simulink model "midterm_block_diagram"  (R2025b)
settings: Solver=VariableStepAuto  StartTime=0.0  StopTime=10.0  RelTol=1e-3
model workspace (MAT data in the model file):
  L_hover = 1
  M_hover = 1
  T_hover = 1
  k1 = 1
  k2 = 1
  k3 = 1
  k4 = 1
  k5 = 1
  x_ref = 1
  y_ref = 1
  z_ref = 1
values from neighbouring files (symbols this model uses):
  K = lqr(A, B, Q, R)    [altitude_control.m]    (also in forward_position_control.m; kalman_filtering.m = P_minus * Cd' / S; lateral_position_control.m; matlab.mat = [0.000497379272644 -0.00135191457606 0.000112708319641 -7.98)
settings Model: Creator=toby0830  LastModifiedBy=tobys

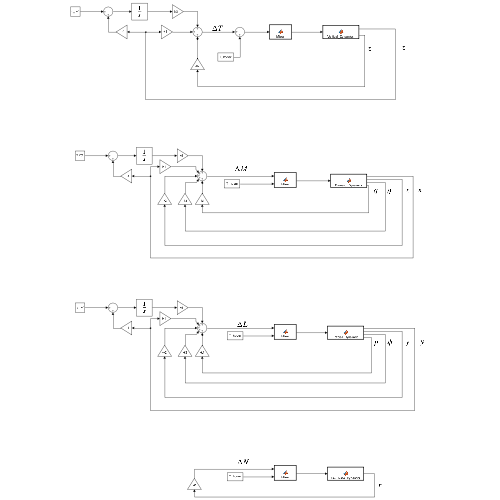
[thumbnail: Simulink's stored preview of the top-level diagram]
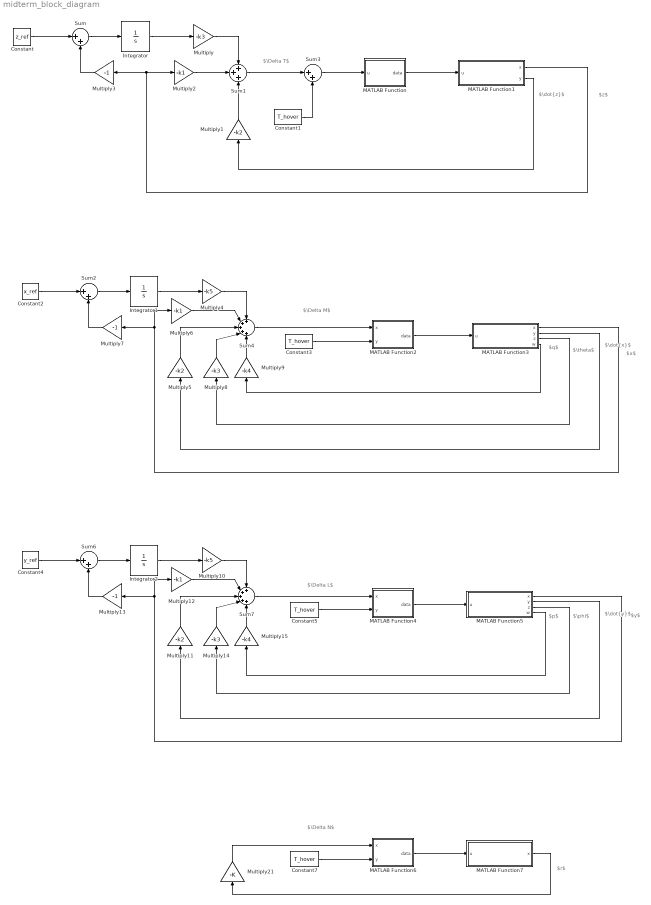
== system midterm_block_diagram ==
  note: $z$
  note: $\dot{x}$
  note: $x$
  note: $\theta$
  note: $q$
  note: $\Delta M$
  note: $\dot{z}$
  note: $\dot{y}$
  note: $y$
  note: $p$
  note: $\Delta L$
  note: $\phi$
  note: $r$
  note: $\Delta N$
  note: $\Delta T$
  Constant : Constant  Value=z_ref
  Constant{1,3,5,7} (4 alike) : Constant  Value=T_hover
  Constant2 : Constant  Value=x_ref
  Constant4 : Constant  Value=y_ref
  Integrator : Integrator
  Integrator1 : Integrator
  Integrator2 : Integrator
  MATLAB Function : MATLAB Function  TreatAsAtomicUnit=on
  MATLAB Function1 : MATLAB Function  TreatAsAtomicUnit=on
  MATLAB Function2 : MATLAB Function  TreatAsAtomicUnit=on
  MATLAB Function3 : MATLAB Function  TreatAsAtomicUnit=on
  MATLAB Function4 : MATLAB Function  TreatAsAtomicUnit=on
  MATLAB Function5 : MATLAB Function  TreatAsAtomicUnit=on
  MATLAB Function6 : MATLAB Function  TreatAsAtomicUnit=on
  MATLAB Function7 : MATLAB Function  TreatAsAtomicUnit=on
  Multiply : Gain  Gain=-k3
  Multiply1 : Gain  Gain=-k2
  Multiply10 : Gain  Gain=-k5
  Multiply11 : Gain  Gain=-k2
  Multiply12 : Gain  Gain=-k1
  Multiply13 : Gain  Gain=-1
  Multiply14 : Gain  Gain=-k3
  Multiply15 : Gain  Gain=-k4
  Multiply2 : Gain  Gain=-k1
  Multiply21 : Gain  Gain=-K
  Multiply3 : Gain  Gain=-1
  Multiply4 : Gain  Gain=-k5
  Multiply5 : Gain  Gain=-k2
  Multiply6 : Gain  Gain=-k1
  Multiply7 : Gain  Gain=-1
  Multiply8 : Gain  Gain=-k3
  Multiply9 : Gain  Gain=-k4
  Sum{,2..3,6} (4 alike) : Sum  Inputs=|++
  Sum1 : Sum  Inputs=+++
  Sum4 : Sum  Inputs=+++++
  Sum7 : Sum  Inputs=+++++
  wires:
  Constant/1 -> Sum/1
  Sum/1 -> Integrator/1
  Integrator/1 -> Multiply/1
  Multiply/1 -> Sum1/1
  Sum1/1 -> Sum3/1
  Constant1/1 -> Sum3/2
  Sum3/1 -> MATLAB Function/1(u)
  MATLAB Function/1(data) -> MATLAB Function1/1(u)
  MATLAB Function1/2(y) -> Multiply1/1
  MATLAB Function1/1(x) -> Multiply3/1, Multiply2/1
  Multiply2/1 -> Sum1/2
  Multiply1/1 -> Sum1/3
  Multiply3/1 -> Sum/2
  Multiply4/1 -> Sum4/1
  MATLAB Function3/2(y) -> Multiply5/1
  Constant2/1 -> Sum2/1
  Multiply7/1 -> Sum2/2
  Integrator1/1 -> Multiply4/1
  Sum2/1 -> Integrator1/1
  Constant3/1 -> MATLAB Function2/2(y)
  MATLAB Function3/1(x) -> Multiply7/1, Multiply6/1
  Multiply5/1 -> Sum4/3
  Multiply6/1 -> Sum4/2
  MATLAB Function2/1(data) -> MATLAB Function3/1(u)
  MATLAB Function3/3(z) -> Multiply8/1
  MATLAB Function3/4(w) -> Multiply9/1
  Multiply8/1 -> Sum4/4
  Multiply9/1 -> Sum4/5
  MATLAB Function5/3(z) -> Multiply14/1
  Multiply11/1 -> Sum7/3
  MATLAB Function5/1(x) -> Multiply13/1, Multiply12/1
  Multiply13/1 -> Sum6/2
  Integrator2/1 -> Multiply10/1
  Sum6/1 -> Integrator2/1
  Multiply14/1 -> Sum7/4
  MATLAB Function4/1(data) -> MATLAB Function5/1(u)
  MATLAB Function5/2(y) -> Multiply11/1
  Multiply15/1 -> Sum7/5
  MATLAB Function5/4(w) -> Multiply15/1
  Sum7/1 -> MATLAB Function4/1(x)
  Multiply10/1 -> Sum7/1
  Multiply12/1 -> Sum7/2
  Constant4/1 -> Sum6/1
  Sum4/1 -> MATLAB Function2/1(x)
  Constant5/1 -> MATLAB Function4/2(y)
  MATLAB Function6/1(data) -> MATLAB Function7/1(u)
  Constant7/1 -> MATLAB Function6/2(y)
  Multiply21/1 -> MATLAB Function6/1(x)
  MATLAB Function7/1(x) -> Multiply21/1

== matlab function midterm_block_diagram/MATLAB Function1 ==
  data: u input; x output; y output
function [x,y]= Vertical_Dynamics(u)

y = u;

== matlab function midterm_block_diagram/MATLAB Function ==
  data: u input; data output
function data = Mixer(u)

y = u;

== matlab function midterm_block_diagram/MATLAB Function2 ==
  data: x input; data output; y input
function data = Mixer(x,y)

y = u;

== matlab function midterm_block_diagram/MATLAB Function3 ==
  data: u input; x output; y output; z output; w output
function [x,y,z,w]= Forward_Dynamics(u)

y = u;

== matlab function midterm_block_diagram/MATLAB Function4 ==
  data: x input; data output; y input
function data = Mixer(x,y)

y = u;

== matlab function midterm_block_diagram/MATLAB Function5 ==
  data: u input; x output; y output; z output; w output
function [x,y,z,w]= Lateral_Dynamics(u)

y = u;

== matlab function midterm_block_diagram/MATLAB Function6 ==
  data: x input; data output; y input
function data = Mixer(x,y)

y = u;

== matlab function midterm_block_diagram/MATLAB Function7 ==
  data: u input; x output
function x = Yaw_Rate_Dynamics(u)

y = u;
